simulink model "PIDControl1"  (R2021a)
settings: Solver=ode45  StartTime=0.0  StopTime=10  FixedStep=0.01  RelTol=1e-3  EnableMultiTasking=on
values from neighbouring files (symbols this model uses):
  Alpha_initial = 0*pi/180    (= 0)    [RIP_PID.m]
  Kd_Alpha = 6.5269    [RIP_PID.m]
  Kd_Theta = -1.7400    (= -1.74)    [RIP_PID.m]
  Ki_Alpha = 0    [RIP_PID.m]
  Ki_Theta = -0    (= 0)    [RIP_PID.m]
  Kp_Alpha = 53.8740    (= 53.874)    [RIP_PID.m]
  Kp_Theta = -2.2361    [RIP_PID.m]
  Theta_desired = 0*pi/180    (= 0)    [RIP_PID.m]
  Theta_initial = 20*pi/180    (= 0.349065850399)    [RIP_PID.m]
libraries: simulink_extras x2
settings Model: Creator=iShAn  LastModifiedBy=ACER
settings SolverCC: ConsecutiveZCsStepRelTol=0  MaxConsecutiveZCs=1000000  ZeroCrossControl=EnableAll  ZeroCrossAlgorithm=Adaptive  AlgebraicLoopSolver=TrustRegion
settings DataIOCC: LimitDataPoints=on  SaveFormat=Array  ReturnWorkspaceOutputs=off
settings OptimizationCC: LifeSpan=inf
settings DebuggingCC: SFUnexpectedBacktrackingDiag=warning  SFNoUnconditionalDefaultTransitionDiag=warning  SFExecutionAtInitializationDiag=none  SFMachineParentedDataDiag=warning  ArithmeticOperatorsInVariantConditions=warning
settings HardwareCC: ProdBitPerPointer=32  ProdBitPerSizeT=32  ProdBitPerPtrDiffT=32  ProdLargestAtomicFloat=None  ProdIntDivRoundTo=Undefined  ProdEndianess=Unspecified  ProdWordSize=32  ProdHWDeviceType=32-bit Generic
settings ModelReferenceCC: PropagateSignalLabelsOutOfModel=off
settings SFSimCC: SimUseLocalCustomCode=off  CustomCodeUndefinedFunction=UseInterfaceOnly
settings RTWCC: GenCodeOnly=on  RTWUseLocalCustomCode=off
settings CodeAppCC: StateflowObjectComments=on
settings GRTTargetCC: TargetLangStandard=C89/C90 (ANSI)
settings ConfigComp: CovMetricSettings=dw  CovSaveCumulativeToWorkspaceVar=on  CovSaveSingleToWorkspaceVar=on  CovExternalEMLEnable=off

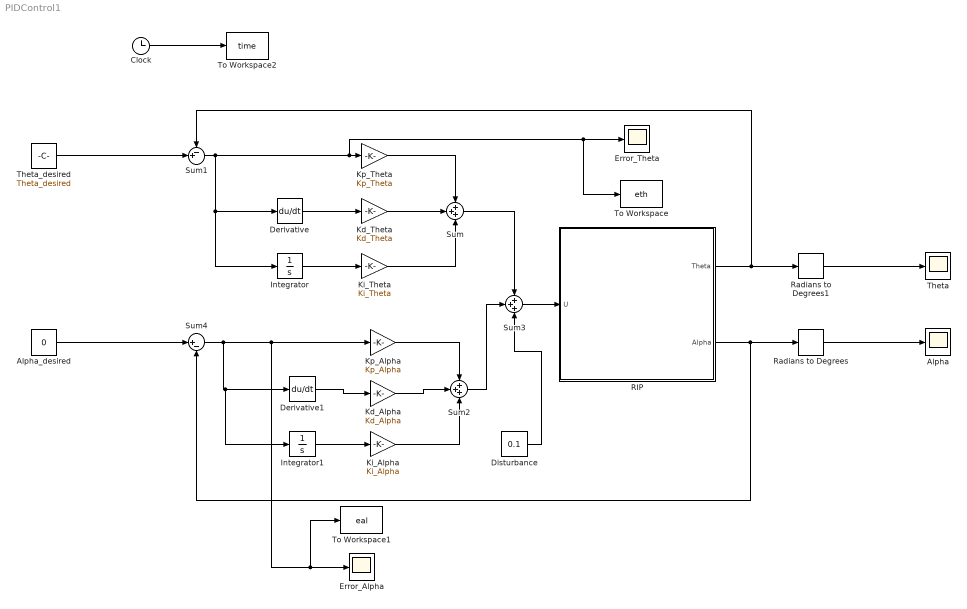
== system PIDControl1 ==
  Alpha : Scope
  Alpha_desired : Constant  Value=0
  Clock : Clock
  Derivative : Derivative
  Derivative1 : Derivative
  Disturbance : Constant  Value=0.1
  Error_Alpha : Scope
  Error_Theta : Scope
  Integrator : Integrator
  Integrator1 : Integrator
  Kd_Alpha : Gain  Gain=Kd_Alpha
  Kd_Theta : Gain  Gain=Kd_Theta
  Ki_Alpha : Gain  Gain=Ki_Alpha
  Ki_Theta : Gain  Gain=Ki_Theta
  Kp_Alpha : Gain  Gain=Kp_Alpha
  Kp_Theta : Gain  Gain=Kp_Theta
  RIP : Subsystem
  Radians to Degrees : simulink_extras/Transformations/Radians to Degrees
  Radians to Degrees1 : simulink_extras/Transformations/Radians to Degrees
  Sum : Sum  Inputs=+++
  Sum1 : Sum  Inputs=-+|
  Sum2 : Sum  Inputs=+++
  Sum3 : Sum  Inputs=+++
  Sum4 : Sum  Inputs=|+-
  Theta : Scope
  Theta_desired : Constant  Value=Theta_desired
  To Workspace : ToWorkspace  VariableName=eth  SampleTime=-1
  To Workspace1 : ToWorkspace  VariableName=eal  SampleTime=-1
  To Workspace2 : ToWorkspace  VariableName=time  SampleTime=-1
  wires:
  Radians to Degrees/1 -> Alpha/1
  Radians to Degrees1/1 -> Theta/1
  RIP/1(Theta) -> Sum1/1, Radians to Degrees1/1
  RIP/2(Alpha) -> Radians to Degrees/1, Sum4/2
  Theta_desired/1 -> Sum1/2
  Sum1/1 -> Integrator/1, Derivative/1, To Workspace/1, Error_Theta/1, Kp_Theta/1
  Derivative/1 -> Kd_Theta/1
  Integrator/1 -> Ki_Theta/1
  Alpha_desired/1 -> Sum4/1
  Derivative1/1 -> Kd_Alpha/1
  Integrator1/1 -> Ki_Alpha/1
  Kd_Theta/1 -> Sum/2
  Kp_Theta/1 -> Sum/1
  Ki_Theta/1 -> Sum/3
  Kd_Alpha/1 -> Sum2/2
  Kp_Alpha/1 -> Sum2/1
  Ki_Alpha/1 -> Sum2/3
  Sum2/1 -> Sum3/2
  Sum3/1 -> RIP/1(U)
  Sum/1 -> Sum3/1
  Sum4/1 -> Integrator1/1, Derivative1/1, To Workspace1/1, Error_Alpha/1, Kp_Alpha/1
  Disturbance/1 -> Sum3/3
  Clock/1 -> To Workspace2/1

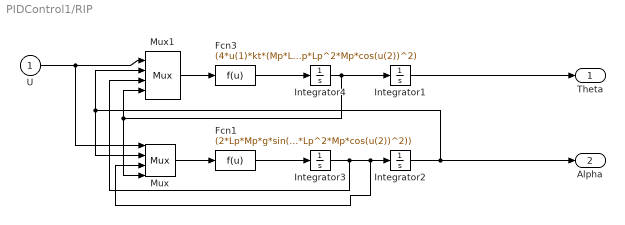
== system PIDControl1/RIP ==
  U : Inport
  Fcn1 : Fcn  Expr=(2*Lp*Mp*g*sin(u(2))*(4*Jr + Lp^2*Mp + 4*Lr^2*Mp - Lp^2*Mp*cos(u(2))^2))/(Lp^4*Mp^2 + 16*Jp*Jr + 4*Lp^2*Lr^2*Mp^2 + 4*Jp*Lp^2*Mp + 16*Jp*Lr^2*Mp + 4*Jr*Lp^2*Mp - Lp^4*Mp^2*cos(u(2))^2 - 4*Lp^2*Lr^2*Mp^2*cos(u(2))^2 - 4*Jp*Lp^2*Mp*cos(u(2))^2) - u(4)*((8*Lp*Lr*Mp*cos(u(2))*((Mp*u(3)*cos(u(2))*sin(u(2))*Lp^2)/2 + Dr + (km*kt)/Rm))/(Lp^4*Mp^2 + 16*Jp*Jr + 4*Lp^2*Lr^2*Mp^2 + 4*Jp*Lp^2*Mp + 16*Jp*Lr^2*Mp + 4*Jr*Lp^2*Mp - Lp^4*Mp^2*cos(u(2))^2 - 4*Lp^2*Lr^2*Mp^2*cos(u(2))^2 - 4*Jp*Lp^2*Mp*cos(u(2))^2) - (Lp^2*Mp*u(4)*cos(u(2))*sin(u(2))*(4*Jr + Lp^2*Mp + 4*Lr^2*Mp - Lp^2*Mp*cos(u(2))^2))/(Lp^4*Mp^2 + 16*Jp*Jr + 4*Lp^2*Lr^2*Mp^2 + 4*Jp*Lp^2*Mp + 16*Jp*Lr^2*Mp + 4*Jr*Lp^2*Mp - Lp^4*Mp^2*cos(u(2))^2 - 4*Lp^2*Lr^2*Mp^2*cos(u(2))^2 - 4*Jp*Lp^2*Mp*cos(u(2))^2)) - u(2)*((4*Dp*(4*Jr + Lp^2*Mp + 4*Lr^2*Mp - Lp^2*Mp*cos(u(2))^2))/(Lp^4*Mp^2 + 16*Jp*Jr + 4*Lp^2*Lr^2*Mp^2 + 4*Jp*Lp^2*Mp + 16*Jp*Lr^2*Mp + 4*Jr*Lp^2*Mp - Lp^4*Mp^2*cos(u(2))^2 - 4*Lp^2*Lr^2*Mp^2*cos(u(2))^2 - 4*Jp*Lp^2*Mp*cos(u(2))^2) + (4*Lp^2*Lr^2*Mp^2*u(3)*cos(u(2))*sin(u(2)))/(Lp^4*Mp^2 + 16*Jp*Jr + 4*Lp^2*Lr^2*Mp^2 + 4*Jp*Lp^2*Mp + 16*Jp*Lr^2*Mp + 4*Jr*Lp^2*Mp - Lp^4*Mp^2*cos(u(2))^2 - 4*Lp^2*Lr^2*Mp^2*cos(u(2))^2 - 4*Jp*Lp^2*Mp*cos(u(2))^2)) + (8*Lp*Lr*Mp*u(1)*kt*cos(u(2)))/(Rm*(Lp^4*Mp^2 + 16*Jp*Jr + 4*Lp^2*Lr^2*Mp^2 + 4*Jp*Lp^2*Mp + 16*Jp*Lr^2*Mp + 4*Jr*Lp^2*Mp - Lp^4*Mp^2*cos(u(2))^2 - 4*Lp^2*Lr^2*Mp^2*cos(u(2))^2 - 4*Jp*Lp^2*Mp*cos(u(2))^2))
  Fcn3 : Fcn  Expr=(4*u(1)*kt*(Mp*Lp^2 + 4*Jp))/(Rm*(Lp^4*Mp^2 + 16*Jp*Jr + 4*Lp^2*Lr^2*Mp^2 + 4*Jp*Lp^2*Mp + 16*Jp*Lr^2*Mp + 4*Jr*Lp^2*Mp - Lp^4*Mp^2*cos(u(2))^2 - 4*Lp^2*Lr^2*Mp^2*cos(u(2))^2 - 4*Jp*Lp^2*Mp*cos(u(2))^2)) - u(4)*((4*(Mp*Lp^2 + 4*Jp)*((Mp*u(3)*cos(u(2))*sin(u(2))*Lp^2)/2 + Dr + (km*kt)/Rm))/(Lp^4*Mp^2 + 16*Jp*Jr + 4*Lp^2*Lr^2*Mp^2 + 4*Jp*Lp^2*Mp + 16*Jp*Lr^2*Mp + 4*Jr*Lp^2*Mp - Lp^4*Mp^2*cos(u(2))^2 - 4*Lp^2*Lr^2*Mp^2*cos(u(2))^2 - 4*Jp*Lp^2*Mp*cos(u(2))^2) - (2*Lp^3*Lr*Mp^2*u(4)*cos(u(2))^2*sin(u(2)))/(Lp^4*Mp^2 + 16*Jp*Jr + 4*Lp^2*Lr^2*Mp^2 + 4*Jp*Lp^2*Mp + 16*Jp*Lr^2*Mp + 4*Jr*Lp^2*Mp - Lp^4*Mp^2*cos(u(2))^2 - 4*Lp^2*Lr^2*Mp^2*cos(u(2))^2 - 4*Jp*Lp^2*Mp*cos(u(2))^2)) - u(2)*((8*Dp*Lp*Lr*Mp*cos(u(2)))/(Lp^4*Mp^2 + 16*Jp*Jr + 4*Lp^2*Lr^2*Mp^2 + 4*Jp*Lp^2*Mp + 16*Jp*Lr^2*Mp + 4*Jr*Lp^2*Mp - Lp^4*Mp^2*cos(u(2))^2 - 4*Lp^2*Lr^2*Mp^2*cos(u(2))^2 - 4*Jp*Lp^2*Mp*cos(u(2))^2) + (2*Lp*Lr*Mp*u(3)*sin(u(2))*(Mp*Lp^2 + 4*Jp))/(Lp^4*Mp^2 + 16*Jp*Jr + 4*Lp^2*Lr^2*Mp^2 + 4*Jp*Lp^2*Mp + 16*Jp*Lr^2*Mp + 4*Jr*Lp^2*Mp - Lp^4*Mp^2*cos(u(2))^2 - 4*Lp^2*Lr^2*Mp^2*cos(u(2))^2 - 4*Jp*Lp^2*Mp*cos(u(2))^2)) + (4*Lp^2*Lr*Mp^2*g*cos(u(2))*sin(u(2)))/(Lp^4*Mp^2 + 16*Jp*Jr + 4*Lp^2*Lr^2*Mp^2 + 4*Jp*Lp^2*Mp + 16*Jp*Lr^2*Mp + 4*Jr*Lp^2*Mp - Lp^4*Mp^2*cos(u(2))^2 - 4*Lp^2*Lr^2*Mp^2*cos(u(2))^2 - 4*Jp*Lp^2*Mp*cos(u(2))^2)
  Integrator1 : Integrator  InitialCondition=Theta_initial
  Integrator2 : Integrator  InitialCondition=Alpha_initial
  Integrator3 : Integrator
  Integrator4 : Integrator
  Mux : Mux
  Mux1 : Mux
  Theta : Outport
  Alpha : Outport  Port=2
  wires:
  Integrator1/1 -> Theta/1
  Mux1/1 -> Fcn3/1
  Fcn3/1 -> Integrator4/1
  Fcn1/1 -> Integrator3/1
  Mux/1 -> Fcn1/1
  Integrator4/1 -> Integrator1/1, Mux/4, Mux1/4
  U/1 -> Mux1/1, Mux/1
  Integrator3/1 -> Mux/3, Integrator2/1, Mux1/3
  Integrator2/1 -> Alpha/1, Mux/2, Mux1/2
